simulink model "qpswnymf"  (Simulink 5.0)
settings: Solver=ode45  StartTime=0.0  StopTime=999999  MaxStep=0.05  MinStep=0.000001  RelTol=1e-6  AbsTol=1e-6
values from neighbouring files (symbols this model uses):
  den = real(poly(p(v:v+1)))    [bwthui.m]    (also in rcosfltk.m = 3)
  num = real(poly(z(index)))    [bwthui.m]    (also in rcosfltk.m = 0.5)
undefined symbols (not defined in the file or in its folder): eyediasi, eyesampl, sbiterr
libraries: librnew x1
CloseFcn:
  | closemodcross
settings Model: Creator=gerhard  LastModifiedBy=bauch  ExtModeAutoUpdateStatusClock=off  SaveTime=off  SaveOutput=off  BlockReductionOpt=off  BooleanDataType=off

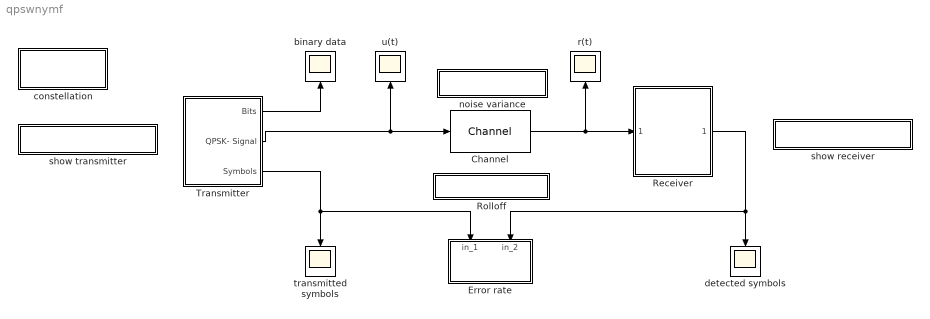
== system qpswnymf ==
  Channel : librnew/Channel  m=0  variance=0.001  s=12345
  Error rate : Subsystem  Orientation=down  LoadFcn=sbiterr([],[],[],'LoadBlock')  StartFcn=sbiterr([],[],[],'Start')  StopFcn=sbiterr([],[],[],'Stop')  mask(Symbol/bit error counter){@1=2, @2=10, @3=12, @4=1}
      mask prompts: @1 "Bit per symbol:"; @2 "Number of digits on display:"; @3 "Delay between 1st port and 2nd port:"; @4 "Sample time (sec):"
      mask help: Use the input data from the 1st port as the reference signal to detect the number of errors and error rate of the 2nd signal.
      mask init:
      | K=@1;num_lin=@2;TDelay=@3;Sample=@4;
      settings: CopyFcn=sbiterr([],[],[],'CopyBlock')  DeleteFcn=sbiterr([],[],[],'DeleteBlock')  NameChangeFcn=sbiterr([],[],[],'NameChange')
      mask Help: The signal from the first port must be a scalar. The second input port can be a vector with a delay to the first port signal. The comparison happens only at the sampling point.
      mask Display: disp('Error\nmeter')
  Receiver : Subsystem
  Rolloff : Subsystem
      settings: OpenFcn=setrloff
      mask Type: rolloff
      mask Display: disp('Rolloff-Factor')
  Transmitter : Subsystem
  binary data : Scope
      settings: Orientation=up  TimeRange=25.000000  YMin=-3  YMax=3  DataFormat=Array
  constellation : Subsystem
      settings: OpenFcn=cplotpsk(4)
      mask Type: constellation
      mask Display: disp('Signal Space \n Constellation')
  detected symbols : Scope
      settings: Orientation=down  TimeRange=25.000000  YMin=-3  YMax=3  DataFormat=Array
  noise variance : Subsystem
      settings: OpenFcn=setnoise
      mask Type: noise
      mask Display: disp('Noise variance')
  r(t) : Scope
      settings: Orientation=up  TimeRange=25.000000  YMin=-1.5  YMax=1.5  DataFormat=Array
  show receiver : Subsystem
      settings: OpenFcn=showrec
      mask Type: open
      mask Display: disp('Receiver')
  show transmitter : Subsystem
      settings: OpenFcn=showtra
      mask Type: open
      mask Display: disp('Transmitter')
  transmitted symbols : Scope
      settings: Orientation=down  TimeRange=25.000000  YMin=-3  YMax=3  DataFormat=Array
  u(t) : Scope
      settings: Orientation=up  TimeRange=25.000000  YMin=-1.5  YMax=1.5  DataFormat=Array
  wires:
  Transmitter/2(QPSK- Signal) -> u(t)/1, Channel/1
  Transmitter/3(Symbols) -> transmitted symbols/1, Error rate/1(in_1)
  Transmitter/1(Bits) -> binary data/1
  Channel/1 -> Receiver/1(noisy QPSK- signal), r(t)/1
  Receiver/1(detected bits) -> detected symbols/1, Error rate/2(in_2)

== system qpswnymf/Error rate ==
  in_1 : Inport
  in_2 : Inport  Port=2
  Mux : Mux  Inputs=2
  S-function : S-Function  FunctionName=sbiterr  Parameters=num_lin, K, TDelay, Sample
  wires:
  Mux/1 -> S-function/1
  in_1/1 -> Mux/1
  in_2/1 -> Mux/2

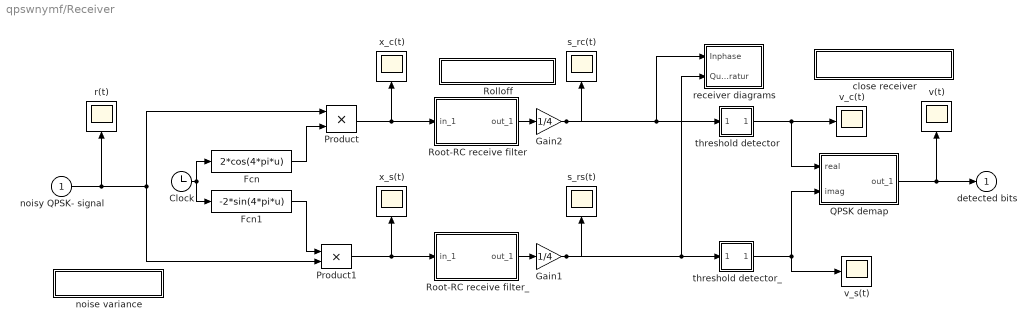
== system qpswnymf/Receiver ==
  noisy QPSK- signal : Inport
  Clock : Clock
      settings: Decimation=10
  Fcn : Fcn  Expr=2*cos(4*pi*u)
  Fcn1 : Fcn  Expr=-2*sin(4*pi*u)
  Gain1 : Gain  Gain=1/4  SaturateOnIntegerOverflow=on
  Gain2 : Gain  Gain=1/4  SaturateOnIntegerOverflow=on
  Product : Product  SaturateOnIntegerOverflow=on  InputSameDT=on
  Product1 : Product  SaturateOnIntegerOverflow=on  InputSameDT=on
  QPSK demap : Subsystem  mask(MPSK demapping){N=[4], A=[sqrt(2)], P=[pi/4], td=1}
      mask prompts: N "Number of symbols on each circle NIC::"; A "Radii for each circle RIC:"; P "Phase shift on each circle PIC (rad):"; td "Symbol interval and offset (sec):"
      mask help:
      | Reverse the QASK map. Input in-phase
      | and quadrature components from the
      | two inputs. Output demapped signal.
      mask init:
      | y1=apkconst(N,A,P);y2=imag(y1);y1=real(y1);
      mask Help: This block demaps a QASK mapped signal using circle constellation. You can place this block after a QAM demodulation block. The circle constellation is defined in NIC, RIC, and PIC. The symbol interval can be a two elements vector with the first element being offset. The default offset is zero. Use function MODMAP to view the constellation.
      mask Display: disp('MPSK\ndemapping')
  Rolloff : Subsystem
      settings: OpenFcn=setrloff
      mask Type: rolloff
      mask Display: disp('Rolloff-Factor')
  Root-RC receive filter : Subsystem  mask(R-C filter){@1=1, @2=.05, @3=.5, @4=6, @5='FIR/Sqrt', @6=0}
      mask prompts: @1 "Symbol interval (sec):"; @2 "Computation sampling time (sec):"; @3 "Filter rolloff factor:"; @4 "Delay step (integer to multiply symbol interval):"; @5 "Filter type (FIR or IIR) / (Normal or Sqrt):"; @6 "With or without sinc filter (1 or 0, suggest 1):"
      mask help: Design a raised cosine filter and use it to filter the input signal.
      mask init:
      | td=@1;if length(td)>1,off=td(2);td=td(1);else,off=0;end;ts=@2;R=@3;delay=@4;fil=@5;[num,den]=rcosine(1/td(1),1/ts(1),fil,R,delay);x=@6/2;
      mask Help: This block designs a raised cosine filter using the specified parameter. The filter is used to filter the input signal. You can optionally use the sinc filter in the filtering computation.
      mask Display: disp('R-C\nfilter')
  Root-RC receive filter_ : Subsystem  mask(R-C filter){@1=1, @2=.05, @3=.5, @4=6, @5='FIR/Sqrt', @6=0}
      mask prompts: @1 "Symbol interval (sec):"; @2 "Computation sampling time (sec):"; @3 "Filter rolloff factor:"; @4 "Delay step (integer to multiply symbol interval):"; @5 "Filter type (FIR or IIR) / (Normal or Sqrt):"; @6 "With or without sinc filter (1 or 0, suggest 1):"
      mask help: Design a raised cosine filter and use it to filter the input signal.
      mask init:
      | td=@1;if length(td)>1,off=td(2);td=td(1);else,off=0;end;ts=@2;R=@3;delay=@4;fil=@5;[num,den]=rcosine(1/td(1),1/ts(1),fil,R,delay);x=@6/2;
      mask Help: This block designs a raised cosine filter using the specified parameter. The filter is used to filter the input signal. You can optionally use the sinc filter in the filtering computation.
      mask Display: disp('R-C\nfilter')
  close receiver : Subsystem
      settings: OpenFcn=closerec
      mask Type: close
      mask Display: disp('close receiver')
  noise variance : Subsystem
      settings: OpenFcn=setnoise
      mask Type: noise
      mask Display: disp('Noise variance')
  r(t) : Scope
      settings: Orientation=up  TimeRange=25.000000  YMin=-1.500000  YMax=1.500000  DataFormat=Array
  receiver diagrams : Subsystem  mask(2D-Diagrams){starttime=12, anzahl=40, offset=0}
      mask prompts: starttime "Plot start time:"; anzahl "Samples per time slot (2*T):"; offset "Decision offset:"
      mask help: Eye pattern, signal space trajectory and scatter plot
      mask init:
      | [x, y] = srcsicon(10);
      mask Display: plot(0,0,100,100,x,y)
  s_rc(t) : Scope
      settings: Orientation=up  TimeRange=25.000000  YMin=-1.500000  YMax=1.500000  DataFormat=Array
  s_rs(t) : Scope
      settings: Orientation=up  TimeRange=25.000000  YMin=-1.500000  YMax=1.500000  DataFormat=Array
  threshold detector : Subsystem
      mask Type: Sign
      mask Description: y = sign(x)
      mask Help: Sign Function:\n\t\t\ty = 1 if x > 0\n\t\t\ty = 0 if x = 0\n\t\t\ty = -1 if x < 0
      mask Display: plot(-50,-50,50,50,[-50,50],[0,0],[0,0],[-50,50],[-40,0],[-30,-30],[0,40],[30,30])
  threshold detector_ : Subsystem
      mask Type: Sign
      mask Description: y = sign(x)
      mask Help: Sign Function:\n\t\t\ty = 1 if x > 0\n\t\t\ty = 0 if x = 0\n\t\t\ty = -1 if x < 0
      mask Display: plot(-50,-50,50,50,[-50,50],[0,0],[0,0],[-50,50],[-40,0],[-30,-30],[0,40],[30,30])
  v(t) : Scope
      settings: Orientation=up  TimeRange=25.000000  YMin=-3.000000  YMax=3.000000  DataFormat=Array
  v_c(t) : Scope
      settings: TimeRange=25.000000  YMin=-1.500000  YMax=1.500000  DataFormat=Array
  v_s(t) : Scope
      settings: TimeRange=25.000000  YMin=-1.500000  YMax=1.500000  DataFormat=Array
  x_c(t) : Scope
      settings: Orientation=up  TimeRange=25.000000  YMin=-1.500000  YMax=1.500000  DataFormat=Array
  x_s(t) : Scope
      settings: Orientation=up  TimeRange=25.000000  YMin=-1.500000  YMax=1.500000  DataFormat=Array
  detected bits : Outport
  wires:
  Clock/1 -> Fcn/1, Fcn1/1
  Product/1 -> Root-RC receive filter/1(in_1), x_c(t)/1
  Product1/1 -> Root-RC receive filter_/1(in_1), x_s(t)/1
  noisy QPSK- signal/1 -> r(t)/1, Product/1, Product1/2
  Fcn1/1 -> Product1/1
  Fcn/1 -> Product/2
  Root-RC receive filter/1(out_1) -> Gain2/1
  Root-RC receive filter_/1(out_1) -> Gain1/1
  Gain2/1 -> s_rc(t)/1, receiver diagrams/1(Inphase), threshold detector/1(in_1)
  Gain1/1 -> s_rs(t)/1, receiver diagrams/2(Quadratur), threshold detector_/1(in_1)
  QPSK demap/1(out_1) -> detected bits/1, v(t)/1
  threshold detector/1(out_1) -> QPSK demap/1(real), v_c(t)/1
  threshold detector_/1(out_1) -> QPSK demap/2(imag), v_s(t)/1

== system qpswnymf/Rolloff ==

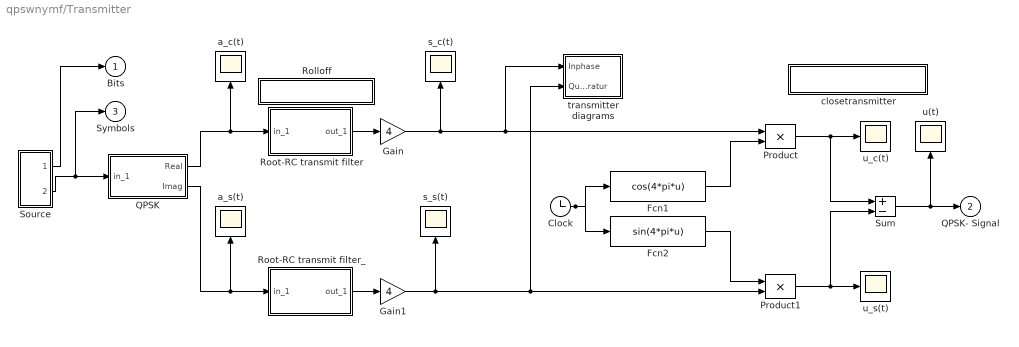
== system qpswnymf/Transmitter ==
  Clock : Clock
      settings: Decimation=10
  Fcn1 : Fcn  Expr=cos(4*pi*u)
  Fcn2 : Fcn  Expr=sin(4*pi*u)
  Gain : Gain  Gain=4  SaturateOnIntegerOverflow=on
  Gain1 : Gain  Gain=4  SaturateOnIntegerOverflow=on
  Product : Product  SaturateOnIntegerOverflow=on  InputSameDT=on
  Product1 : Product  SaturateOnIntegerOverflow=on  InputSameDT=on
  QPSK : Subsystem  mask(MPSK){N=[4], A=[sqrt(2)], P=[pi/4], td=1}
      mask prompts: N "Number of symbols in each circle NIC:"; A "Radii in each circle RIC:"; P "Phase shift in each circle PIC (rad):"; td "Symbol interval and offset (sec):"
      mask help: QASK mapping with circle constellation. The constellation is defined in NIC, RIC and PIC.
      mask init:
      | y1=apkconst(N,A,P);y1=[y1;y1];y1=y1(:);y2=imag(y1);y1=real(y1);x=[-sum(N) 1:sum(N)-1;1:sum(N)-1 10*sum(N)]-.5;x=x(:);
      mask Help: This block maps a digital signal onto in-phase and quadratic components, which are outputs in the first and second output port respectively. The circle constellation is defined in NIC, RIC, and PIC. The input symbol interval can be a two-element vector with the second element being offset. The default value offset is 0. Use the MODMAP function to see the constellation.
      mask Display: disp('MPSK\nmapping')
  Rolloff : Subsystem
      settings: OpenFcn=setrloff
      mask Type: rolloff
      mask Display: disp('Rolloff-Factor')
  Root-RC transmit filter : Subsystem  mask(R-C filter){@1=1, @2=.05, @3=.5, @4=6, @5='FIR/Sqrt', @6=1}
      mask prompts: @1 "Symbol interval (sec):"; @2 "Computation sampling time (sec):"; @3 "Filter rolloff factor:"; @4 "Delay step (integer to multiply symbol interval):"; @5 "Filter type (FIR or IIR) / (Normal or Sqrt):"; @6 "With or without sinc filter (1 or 0, suggest 1):"
      mask help: Design a raised cosine filter and use it to filter the input signal.
      mask init:
      | td=@1;if length(td)>1,off=td(2);td=td(1);else,off=0;end;ts=@2;R=@3;delay=@4;fil=@5;[num,den]=rcosine(1/td(1),1/ts(1),fil,R,delay);x=@6/2;
      mask Help: This block designs a raised cosine filter using the specified parameter. The filter is used to filter the input signal. You can optionally use the sinc filter in the filtering computation.
      mask Display: disp('R-C\nfilter')
  Root-RC transmit filter_ : Subsystem  mask(R-C filter){@1=1, @2=.05, @3=.5, @4=6, @5='FIR/Sqrt', @6=1}
      mask prompts: @1 "Symbol interval (sec):"; @2 "Computation sampling time (sec):"; @3 "Filter rolloff factor:"; @4 "Delay step (integer to multiply symbol interval):"; @5 "Filter type (FIR or IIR) / (Normal or Sqrt):"; @6 "With or without sinc filter (1 or 0, suggest 1):"
      mask help: Design a raised cosine filter and use it to filter the input signal.
      mask init:
      | td=@1;if length(td)>1,off=td(2);td=td(1);else,off=0;end;ts=@2;R=@3;delay=@4;fil=@5;[num,den]=rcosine(1/td(1),1/ts(1),fil,R,delay);x=@6/2;
      mask Help: This block designs a raised cosine filter using the specified parameter. The filter is used to filter the input signal. You can optionally use the sinc filter in the filtering computation.
      mask Display: disp('R-C\nfilter')
  Source : Subsystem
  Sum : Sum  Inputs=+-  SaturateOnIntegerOverflow=on  InputSameDT=on
  a_c(t) : Scope
      settings: Orientation=up  TimeRange=25.000000  YMin=-1.500000  YMax=1.500000  DataFormat=Array
  a_s(t) : Scope
      settings: Orientation=up  TimeRange=25.000000  YMin=-1.500000  YMax=1.500000  DataFormat=Array
  closetransmitter : Subsystem
      settings: OpenFcn=closetra
      mask Type: close
      mask Display: disp('Close transmitter')
  s_c(t) : Scope
      settings: Orientation=up  TimeRange=25.000000  YMin=-1.500000  YMax=1.500000  DataFormat=Array
  s_s(t) : Scope
      settings: Orientation=up  TimeRange=25.000000  YMin=-1.500000  YMax=1.500000  DataFormat=Array
  transmitter diagrams : Subsystem  mask(2D-Diagrams){starttime=6, anzahl=40, offset=0}
      mask prompts: starttime "Plot start time:"; anzahl "Samples per time slot (2*T):"; offset "Decision offset:"
      mask help: Eye pattern, signal space trajectory and scatter plot
      mask init:
      | [x, y] = srcsicon(10);
      mask Display: plot(0,0,100,100,x,y)
  u(t) : Scope
      settings: Orientation=up  TimeRange=25.000000  YMin=-1.500000  YMax=1.500000  DataFormat=Array
  u_c(t) : Scope
      settings: TimeRange=25.000000  YMin=-1.500000  YMax=1.500000  DataFormat=Array
  u_s(t) : Scope
      settings: TimeRange=25.000000  YMin=-1.500000  YMax=1.500000  DataFormat=Array
  Bits : Outport
  QPSK- Signal : Outport  Port=2
  Symbols : Outport  Port=3
  wires:
  QPSK/2(Imag) -> Root-RC transmit filter_/1(in_1), a_s(t)/1
  QPSK/1(Real) -> Root-RC transmit filter/1(in_1), a_c(t)/1
  Source/2(Symbol) -> QPSK/1(in_1), Symbols/1
  Product1/1 -> u_s(t)/1, Sum/2
  Product/1 -> u_c(t)/1, Sum/1
  Gain/1 -> s_c(t)/1, Product/1, transmitter diagrams/1(Inphase)
  Gain1/1 -> s_s(t)/1, Product1/2, transmitter diagrams/2(Quadratur)
  Root-RC transmit filter_/1(out_1) -> Gain1/1
  Root-RC transmit filter/1(out_1) -> Gain/1
  Clock/1 -> Fcn2/1, Fcn1/1
  Fcn1/1 -> Product/2
  Fcn2/1 -> Product1/1
  Sum/1 -> u(t)/1, QPSK- Signal/1
  Source/1(binary) -> Bits/1

== system qpswnymf/constellation ==

== system qpswnymf/noise variance ==

== system qpswnymf/show receiver ==

== system qpswnymf/show transmitter ==

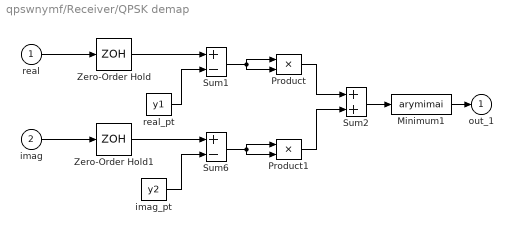
== system qpswnymf/Receiver/QPSK demap ==
  real : Inport
  imag : Inport  Port=2
  Minimum1 : S-Function  FunctionName=arymimai  Parameters='min'
  Product : Product  SaturateOnIntegerOverflow=on  InputSameDT=on
  Product1 : Product  SaturateOnIntegerOverflow=on  InputSameDT=on
  Sum1 : Sum  Inputs=+-  SaturateOnIntegerOverflow=on  InputSameDT=on
  Sum2 : Sum  SaturateOnIntegerOverflow=on  InputSameDT=on
  Sum6 : Sum  Inputs=+-  SaturateOnIntegerOverflow=on  InputSameDT=on
  Zero-Order Hold : ZeroOrderHold  SampleTime=td
  Zero-Order Hold1 : ZeroOrderHold  SampleTime=td
  imag_pt : Constant  Value=y2
  real_pt : Constant  Value=y1
  out_1 : Outport
  wires:
  Minimum1/1 -> out_1/1
  Sum2/1 -> Minimum1/1
  Product1/1 -> Sum2/2
  Product/1 -> Sum2/1
  Sum6/1 -> Product1/2, Product1/1
  Sum1/1 -> Product/2, Product/1
  imag_pt/1 -> Sum6/2
  Zero-Order Hold1/1 -> Sum6/1
  Zero-Order Hold/1 -> Sum1/1
  real_pt/1 -> Sum1/2
  imag/1 -> Zero-Order Hold1/1
  real/1 -> Zero-Order Hold/1

== system qpswnymf/Receiver/Rolloff ==

== system qpswnymf/Receiver/Root-RC receive filter ==
  in_1 : Inport
  Filter : DiscreteFilter  Numerator=num  Denominator=den  SampleTime=ts
  Memory Impulse : Subsystem  mask(Impulse){@1=ts, @2=x}
      mask prompts: @1 "Holding time:"; @2 "Threshold for clock pulse:"
      mask help: 1/sinc filter:
      mask init:
      | ts=@1;thr=@2;x=thr>0;
      mask Help: When the threshold is greater than zero, this block outputs an impulse signal, which begins at the raising edge of the second input and lasts the holding time. The impulse holds a constant amplitude, which equals the amplitude of the first input at the begining of the impulse. A clock raising edge will trigger next impulse. When the threshold is less or equal to zero, this block faithfully outputs the first input.
      mask Display: disp('1/sinc')
  Pulses deivide same sample time1 : Subsystem  mask(Pulse generator){@1=td, @2=1, @3=off}
      mask prompts: @1 "Sample time (scalar, sec):"; @2 "Divider (integer vector):"; @3 "Offset (have same dimension as Divider:"
      mask help: Vector pulses with sample rate of each pulse as Sample_time ./Divider.
      mask init:
      | samp_time=@1;out_divid=@2;offset=@3;
      mask Help: This block generator a vector pulses. The output length is the same as the vector defined in "Divider". The ith element of the output has the sample time Sample_time/Divider(i). All elements in "Divider" must be integers.
      mask Display: disp('Vector\nPulse')
  out_1 : Outport
  wires:
  Pulses deivide same sample time1/1(Outport) -> Memory Impulse/2(in_2)
  Memory Impulse/1(out_1) -> Filter/1
  in_1/1 -> Memory Impulse/1(in_1)
  Filter/1 -> out_1/1

== system qpswnymf/Receiver/Root-RC receive filter_ ==
  in_1 : Inport
  Filter : DiscreteFilter  Numerator=num  Denominator=den  SampleTime=ts
  Memory Impulse : Subsystem  mask(Impulse){@1=ts, @2=x}
      mask prompts: @1 "Holding time:"; @2 "Threshold for clock pulse:"
      mask help: 1/sinc filter:
      mask init:
      | ts=@1;thr=@2;x=thr>0;
      mask Help: When the threshold is greater than zero, this block outputs an impulse signal, which begins at the raising edge of the second input and lasts the holding time. The impulse holds a constant amplitude, which equals the amplitude of the first input at the begining of the impulse. A clock raising edge will trigger next impulse. When the threshold is less or equal to zero, this block faithfully outputs the first input.
      mask Display: disp('1/sinc')
  Pulses deivide same sample time1 : Subsystem  mask(Pulse generator){@1=td, @2=1, @3=off}
      mask prompts: @1 "Sample time (scalar, sec):"; @2 "Divider (integer vector):"; @3 "Offset (have same dimension as Divider:"
      mask help: Vector pulses with sample rate of each pulse as Sample_time ./Divider.
      mask init:
      | samp_time=@1;out_divid=@2;offset=@3;
      mask Help: This block generator a vector pulses. The output length is the same as the vector defined in "Divider". The ith element of the output has the sample time Sample_time/Divider(i). All elements in "Divider" must be integers.
      mask Display: disp('Vector\nPulse')
  out_1 : Outport
  wires:
  Filter/1 -> out_1/1
  in_1/1 -> Memory Impulse/1(in_1)
  Memory Impulse/1(out_1) -> Filter/1
  Pulses deivide same sample time1/1(Outport) -> Memory Impulse/2(in_2)

== system qpswnymf/Receiver/close receiver ==

== system qpswnymf/Receiver/noise variance ==

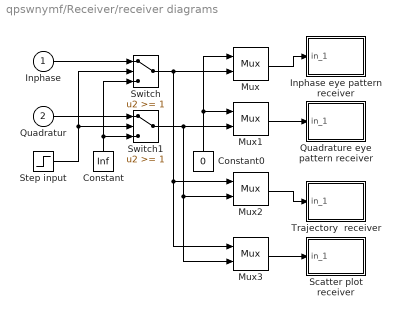
== system qpswnymf/Receiver/receiver diagrams ==
  Inphase : Inport
  Quadratur : Inport  Port=2
  Constant : Constant  Orientation=up  Value=Inf
  Constant0 : Constant  Orientation=up  Value=0
  Inphase eye pattern receiver : Subsystem  LoadFcn=eyesampl([],[],[],'LoadBlock')  StartFcn=eyesampl([],[],[],'Start')  StopFcn=eyesampl([],[],[],'Stop')  mask(Eye-diagram/scatter plot){@1=[2 0 1+offset], @2=[-1.5 1.5], @3=0, @4='w-/r-', @5=0, @6=2/anzahl}
      mask prompts: @1 "[Symbol interval, plot offset, decision point offset]:"; @2 "Lower and upper bound of in-coming signal (1x2 vector):"; @3 "Number of saved traces:"; @4 "Line-type for eye-pattern diagram (0 for no plot):"; @5 "Line-type for scatter plot (0 for no plot):"; @6 "Plot update sample time:"
      mask help: Produce eye-pattern diagram and/or scatter plot.
      mask init:
      | time_range=@1;boundary=@2;kept_length=@3;eye_line=@4;scatter_line=@5;two_d_line=@6;[x,y]=srcsicon(10);
      settings: CopyFcn=eyesampl([],[],[],'CopyBlock')  DeleteFcn=eyesampl([],[],[],'DeleteBlock')  NameChangeFcn=eyesampl([],[],[],'NameChange')
      mask Help: This plot opens one, or two plots by assigning the line type parameters. The scatter plot point is selected by the decision point in the first parameter entry. A decision line is drawn in the eye-pattern diagram. The plot is updated at the plot update sample time point.
      mask Display: plot(0,0,100,100,x,y);
  Mux{,1..3} (4 alike) : Mux  Inputs=2
  Quadrature eye pattern receiver : Subsystem  LoadFcn=eyesampl([],[],[],'LoadBlock')  StartFcn=eyesampl([],[],[],'Start')  StopFcn=eyesampl([],[],[],'Stop')  mask(Eye-diagram/scatter plot){@1=[2 0 1+offset], @2=[-1.5 1.5], @3=0, @4='w-/r-', @5=0, @6=2/anzahl}
      mask prompts: @1 "[Symbol interval, plot offset, decision point offset]:"; @2 "Lower and upper bound of in-coming signal (1x2 vector):"; @3 "Number of saved traces:"; @4 "Line-type for eye-pattern diagram (0 for no plot):"; @5 "Line-type for scatter plot (0 for no plot):"; @6 "Plot update sample time:"
      mask help: Produce eye-pattern diagram and/or scatter plot.
      mask init:
      | time_range=@1;boundary=@2;kept_length=@3;eye_line=@4;scatter_line=@5;two_d_line=@6;[x,y]=srcsicon(10);
      settings: CopyFcn=eyesampl([],[],[],'CopyBlock')  DeleteFcn=eyesampl([],[],[],'DeleteBlock')  NameChangeFcn=eyesampl([],[],[],'NameChange')
      mask Help: This plot opens one, or two plots by assigning the line type parameters. The scatter plot point is selected by the decision point in the first parameter entry. A decision line is drawn in the eye-pattern diagram. The plot is updated at the plot update sample time point.
      mask Display: plot(0,0,100,100,x,y);
  Scatter plot receiver : Subsystem  LoadFcn=eyesampl([],[],[],'LoadBlock')  StartFcn=eyesampl([],[],[],'Start')  StopFcn=eyesampl([],[],[],'Stop')  mask(Eye-diagram/scatter plot){@1=[1 .5 .999], @2=[-1.5 1.5], @3=0, @4=0, @5='b.', @6=[.5 offset]}
      mask prompts: @1 "[Symbol interval, plot offset, decision point offset]:"; @2 "Lower and upper bound of in-coming signal (1x2 vector):"; @3 "Number of saved traces:"; @4 "Line-type for eye-pattern diagram (0 for no plot):"; @5 "Line-type for scatter plot (0 for no plot):"; @6 "Plot update sample time:"
      mask help: Produce eye-pattern diagram and/or scatter plot.
      mask init:
      | time_range=@1;boundary=@2;kept_length=@3;eye_line=@4;scatter_line=@5;two_d_line=@6;[x,y]=srcsicon(10);
      settings: CopyFcn=eyesampl([],[],[],'CopyBlock')  DeleteFcn=eyesampl([],[],[],'DeleteBlock')  NameChangeFcn=eyesampl([],[],[],'NameChange')
      mask Help: This plot opens one, or two plots by assigning the line type parameters. The scatter plot point is selected by the decision point in the first parameter entry. A decision line is drawn in the eye-pattern diagram. The plot is updated at the plot update sample time point.
      mask Display: plot(0,0,100,100,x,y);
  Step input : Step  Time=starttime  SampleTime=1
  Switch : Switch  Threshold=1  SaturateOnIntegerOverflow=on  InputSameDT=on
  Switch1 : Switch  Threshold=1  SaturateOnIntegerOverflow=on  InputSameDT=on
  Trajectory  receiver : Subsystem  LoadFcn=eyediasi([],[],[],'LoadBlock')  StartFcn=eyediasi([],[],[],'Start')  StopFcn=eyediasi([],[],[],'Stop')  mask(Eye-diagram/scatter plot){@1=[2 0 1], @2=[-1.5 1.5], @3=0, @4=0, @5=0, @6='g-'}
      mask prompts: @1 "Eye-pattern plot time frame:"; @2 "Lower and upper bound of in-coming signal (1x2 vector):"; @3 "Number of saved traces:"; @4 "Line-type for eye-pattern diagram (0 for no plot):"; @5 "Line-type for scatter plot (0 for no plot):"; @6 "Line-type for x-y plot (0 for no plot):"
      mask help:
      | Produce eye-pattern diagram/scatter
      | plot/x-y plot with the rising edge of the second input as the decision line.
      mask init:
      | time_range=@1;boundary=@2;kept_length=@3;eye_line=@4;scatter_line=@5;two_d_line=@6;[x,y]=srcsicon(10);[v,w]=trigicon(0,25,get_param(gcb,'orientation'),2);
      settings: CopyFcn=eyediasi([],[],[],'CopyBlock')  DeleteFcn=eyediasi([],[],[],'DeleteBlock')  NameChangeFcn=eyediasi([],[],[],'NameChange')
      mask Help: This plot opens one, two, or three plots by assigning the line type parameters. The scatter plot point is selected by the rising edge of a trigger signal. A decision line is drawn at the rising edge of the trigger signal.
      mask Display: plot(0,0,100,100,x,y,v,w);
  wires:
  Switch/1 -> Mux/2, Mux3/1, Mux2/1
  Switch1/1 -> Mux1/2, Mux3/2, Mux2/2
  Constant0/1 -> Mux1/1, Mux/1
  Quadratur/1 -> Switch1/1
  Inphase/1 -> Switch/1
  Step input/1 -> Switch/2, Switch1/2
  Constant/1 -> Switch/3, Switch1/3
  Mux1/1 -> Quadrature eye pattern receiver/1(in_1)
  Mux/1 -> Inphase eye pattern receiver/1(in_1)
  Mux3/1 -> Scatter plot receiver/1(in_1)
  Mux2/1 -> Trajectory  receiver/1(in_1)

== system qpswnymf/Receiver/threshold detector ==
  in_1 : Inport
  Constant : Constant  Value=0
  Relational Operator : RelationalOperator  Operator=>  InputSameDT=on
  Relational Operator1 : RelationalOperator  Operator=<  InputSameDT=on
  Sum : Sum  Inputs=+-  SaturateOnIntegerOverflow=on  InputSameDT=on
  out_1 : Outport
  wires:
  in_1/1 -> Relational Operator/1, Relational Operator1/1
  Constant/1 -> Relational Operator1/2, Relational Operator/2
  Relational Operator1/1 -> Sum/2
  Relational Operator/1 -> Sum/1
  Sum/1 -> out_1/1

== system qpswnymf/Receiver/threshold detector_ ==
  in_1 : Inport
  Constant : Constant  Value=0
  Relational Operator : RelationalOperator  Operator=>  InputSameDT=on
  Relational Operator1 : RelationalOperator  Operator=<  InputSameDT=on
  Sum : Sum  Inputs=+-  SaturateOnIntegerOverflow=on  InputSameDT=on
  out_1 : Outport
  wires:
  Sum/1 -> out_1/1
  Relational Operator/1 -> Sum/1
  Relational Operator1/1 -> Sum/2
  Constant/1 -> Relational Operator1/2, Relational Operator/2
  in_1/1 -> Relational Operator/1, Relational Operator1/1

== system qpswnymf/Transmitter/QPSK ==
  in_1 : Inport
  Zero-Order Hold1 : ZeroOrderHold  SampleTime=td
  imag part1 : Lookup  InputValues=x  OutputValues=y2  SaturateOnIntegerOverflow=on
  real part : Lookup  InputValues=x  OutputValues=y1  SaturateOnIntegerOverflow=on
  Real : Outport
  Imag : Outport  Port=2
  wires:
  in_1/1 -> Zero-Order Hold1/1
  Zero-Order Hold1/1 -> real part/1, imag part1/1
  real part/1 -> Real/1
  imag part1/1 -> Imag/1

== system qpswnymf/Transmitter/Rolloff ==

== system qpswnymf/Transmitter/Root-RC transmit filter ==
  in_1 : Inport
  Filter : DiscreteFilter  Numerator=num  Denominator=den  SampleTime=ts
  Memory Impulse : Subsystem  mask(Impulse){@1=ts, @2=x}
      mask prompts: @1 "Holding time:"; @2 "Threshold for clock pulse:"
      mask help: 1/sinc filter:
      mask init:
      | ts=@1;thr=@2;x=thr>0;
      mask Help: When the threshold is greater than zero, this block outputs an impulse signal, which begins at the raising edge of the second input and lasts the holding time. The impulse holds a constant amplitude, which equals the amplitude of the first input at the begining of the impulse. A clock raising edge will trigger next impulse. When the threshold is less or equal to zero, this block faithfully outputs the first input.
      mask Display: disp('1/sinc')
  Pulses deivide same sample time1 : Subsystem  mask(Pulse generator){@1=td, @2=1, @3=off}
      mask prompts: @1 "Sample time (scalar, sec):"; @2 "Divider (integer vector):"; @3 "Offset (have same dimension as Divider:"
      mask help: Vector pulses with sample rate of each pulse as Sample_time ./Divider.
      mask init:
      | samp_time=@1;out_divid=@2;offset=@3;
      mask Help: This block generator a vector pulses. The output length is the same as the vector defined in "Divider". The ith element of the output has the sample time Sample_time/Divider(i). All elements in "Divider" must be integers.
      mask Display: disp('Vector\nPulse')
  out_1 : Outport
  wires:
  Pulses deivide same sample time1/1(Outport) -> Memory Impulse/2(in_2)
  Memory Impulse/1(out_1) -> Filter/1
  in_1/1 -> Memory Impulse/1(in_1)
  Filter/1 -> out_1/1

== system qpswnymf/Transmitter/Root-RC transmit filter_ ==
  in_1 : Inport
  Filter : DiscreteFilter  Numerator=num  Denominator=den  SampleTime=ts
  Memory Impulse : Subsystem  mask(Impulse){@1=ts, @2=x}
      mask prompts: @1 "Holding time:"; @2 "Threshold for clock pulse:"
      mask help: 1/sinc filter:
      mask init:
      | ts=@1;thr=@2;x=thr>0;
      mask Help: When the threshold is greater than zero, this block outputs an impulse signal, which begins at the raising edge of the second input and lasts the holding time. The impulse holds a constant amplitude, which equals the amplitude of the first input at the begining of the impulse. A clock raising edge will trigger next impulse. When the threshold is less or equal to zero, this block faithfully outputs the first input.
      mask Display: disp('1/sinc')
  Pulses deivide same sample time1 : Subsystem  mask(Pulse generator){@1=td, @2=1, @3=off}
      mask prompts: @1 "Sample time (scalar, sec):"; @2 "Divider (integer vector):"; @3 "Offset (have same dimension as Divider:"
      mask help: Vector pulses with sample rate of each pulse as Sample_time ./Divider.
      mask init:
      | samp_time=@1;out_divid=@2;offset=@3;
      mask Help: This block generator a vector pulses. The output length is the same as the vector defined in "Divider". The ith element of the output has the sample time Sample_time/Divider(i). All elements in "Divider" must be integers.
      mask Display: disp('Vector\nPulse')
  out_1 : Outport
  wires:
  Pulses deivide same sample time1/1(Outport) -> Memory Impulse/2(in_2)
  Memory Impulse/1(out_1) -> Filter/1
  in_1/1 -> Memory Impulse/1(in_1)
  Filter/1 -> out_1/1

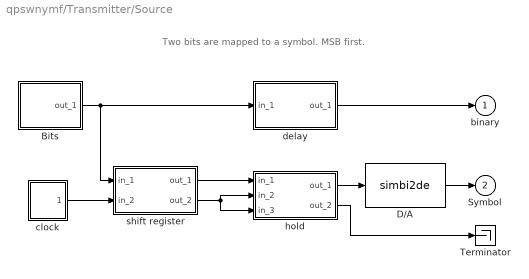
== system qpswnymf/Transmitter/Source ==
  note: Two bits are mapped to a symbol. MSB first.
  Bits : Subsystem  mask(Read from workspace){@1=randint(2000,1,2), @2=.5, @3=1, @4=1}
      mask prompts: @1 "Variable (column_number=block_output_length):"; @2 "Data output sample time (sec):"; @3 "Repeat flag (1: repeat read, 0: output zeros after eof)."; @4 "Initial output:"
      mask help:
      | Read from a workspace variable at
      | sampling time point.
      mask init:
      | var=@1;td=@2;ts=td(1);if (length(td)>=2),off=td(2);else off=0;end;cyc=@3;ini=@4;[x,y]=srcsicon(7);
      mask Help: This block reads from a workspace variable at a given sample time. The column number is the block output vector length. When the simulation reaches the end of the variable (eof), the block will cyclically output from the first row of the variable or output zeros based on the repeat flag entree.
      mask Display: plot(0,0,100,100,x,y);disp('Rd wksp')
  "D/A " : S-Function  FunctionName=simbi2de  Parameters=p  mask(Base M vector to decimal integer){@1=2}
      mask prompts: @1 "Input integer base M:"
      mask help:
      | Convert base M integer with each
      | position in the input vector into scalar decimal output.
      mask init:
      | p=@1;
      mask Help: This block convert the base M vector into scalar decimal integer output. Each element of the input vector is one position of the digit of the base M integer. The 1st element in the input vector contains the 1's position. The 2nd element in the input vector contains the M's position.
      mask Display: disp('Vec to sca\nconverter')
  Terminator : Terminator
  clock : Subsystem  mask(Pulse Generator){@1=.5, @2=.25, @3=1, @4=0}
      mask prompts: @1 "Pulse period (secs):"; @2 "Pulse width:"; @3 "Pulse height:"; @4 "Pulse start time:"
      mask help: Pulse Generator.
      mask init:
      | Ts=@1; du=@2; ht=@3; stt=@4; ini=ones(length(ht),1); st1=rem(stt,Ts); st2=rem(stt+du,Ts);if(Ts<=1.2*du),ini=zeros(length(ht),1);end;
      mask Help: Pulse generator which ensures pulse\ntransitions are hit. Provides a vector of pulses when the height is entered as a vector.\nUnmask to see how it works.
      mask Display: plot(0,0,100,100,[90,75,75,60,60,35,35,20,20,10],[20,20,80,80,20,20,80,80,20,20])
  delay : Subsystem  mask(Multi-step delay){@1=2, @2=.5, @3=0}
      mask prompts: @1 "Delay steps (integer):"; @2 "Sample time (sec):"; @3 "Initial output:"
      mask help: Output is K-step delay of the input signal.
      mask init:
      | n=@1;ts=@2;if length(ts)<2, ts=[ts 0];end;ini=@3;
      mask Help: This block holds the input signal for K steps and then outputs the signal. The delay step cannot be changed during the simulation.
      mask Display: disp('-k\nz   ')
  hold : Subsystem  mask(Triggered buffer down){@1=2, @2=[1 0], @3=[0 0], @4=1, @5=0}
      mask prompts: @1 "Input signal vector size:"; @2 "Initial index (integer vector):"; @3 "Increment for each index (integer vector):"; @4 "Trigger threshold:"; @5 "When index exceed register size, 1: cyclic out, 0: zero out:"
      mask help: Rising edge of the 2nd port triggers 1st port vector signal in. Rising edge of the 3rd port triggers 1st outport signal out.
      mask init:
      | in_size=@1;ini_idx=@2;idx_inc=@3;thrshld=@4;cycl_flag=@5;out_size=length(ini_idx);[v,w]=trigicon(0,25,get_param(gcb,'orientation'),2);[x,y]=trigicon(1,75,get_param(gcb,'orientation'),2);[u,z]=trigicon(0,50,get_param(gcb,'orientation'),2);
      mask Help: The block refreshes its registers with the vector input from the 1st inport at the rising edge of the 2nd inport pulse. The 1st outport outputs the elements of the registers starting with the given initial index. The rising edge of the 3rd inport pulse triggers the 1st output to output the register value with the index increasing the increment value. The second outport outputs a spike pulse when the internal register is refreshed.
      mask Display: plot(0,0,100,100,x,y,v,w,u,z);disp('Buffer dwn')
  shift register : Subsystem  mask(Register-shift){@1=[2 1], @2=1}
      mask prompts: @1 "Delay steps (output length is same as this vector size):"; @2 "Threshold in detecting the rising edge of the pulse:"
      mask help:
      | The rising edge of the 2nd port pulse
      | triggers the block to input the 1st port data and to shift the register.
      mask init:
      | shft_out=@1;thrhld=@2;len_rg=length(@1);[v,w]=trigicon(0,25,get_param(gcb,'orientation'),2);[x,y]=trigicon(1,75,get_param(gcb,'orientation'),2);
      mask Help: This block stores the scalar input signal from the 1st input port at the rising edge of the pulse from the 2nd port. The 1st outport outputs a vector with its size the same as the "Delay steps" entree of this block. The maximum delay is the register size of this block. The second outport outputs a positive pulse when the register is\nrefreshed.
      mask Display: plot(0,0,100,100,x,y,v,w);disp('Reg. shift')
  binary : Outport
  Symbol : Outport  Port=2
  wires:
  hold/2(out_2) -> Terminator/1
  "D/A "/1 -> Symbol/1
  delay/1(out_1) -> binary/1
  shift register/1(out_1) -> hold/1(in_1)
  hold/1(out_1) -> "D/A "/1
  clock/1(out_1) -> shift register/2(in_2)
  shift register/2(out_2) -> hold/2(in_2), hold/3(in_3)
  Bits/1(out_1) -> delay/1(in_1), shift register/1(in_1)

== system qpswnymf/Transmitter/closetransmitter ==

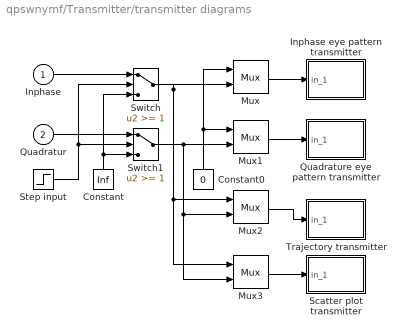
== system qpswnymf/Transmitter/transmitter diagrams ==
  Inphase : Inport
  Quadratur : Inport  Port=2
  Constant : Constant  Orientation=up  Value=Inf
  Constant0 : Constant  Orientation=up  Value=0
  Inphase eye pattern transmitter : Subsystem  LoadFcn=eyesampl([],[],[],'LoadBlock')  StartFcn=eyesampl([],[],[],'Start')  StopFcn=eyesampl([],[],[],'Stop')  mask(Eye-diagram/scatter plot){@1=[2 0 1+offset], @2=[-1.5 1.5], @3=0, @4='w-/r-', @5=0, @6=2/anzahl}
      mask prompts: @1 "[Symbol interval, plot offset, decision point offset]:"; @2 "Lower and upper bound of in-coming signal (1x2 vector):"; @3 "Number of saved traces:"; @4 "Line-type for eye-pattern diagram (0 for no plot):"; @5 "Line-type for scatter plot (0 for no plot):"; @6 "Plot update sample time:"
      mask help: Produce eye-pattern diagram and/or scatter plot.
      mask init:
      | time_range=@1;boundary=@2;kept_length=@3;eye_line=@4;scatter_line=@5;two_d_line=@6;[x,y]=srcsicon(10);
      settings: CopyFcn=eyesampl([],[],[],'CopyBlock')  DeleteFcn=eyesampl([],[],[],'DeleteBlock')  NameChangeFcn=eyesampl([],[],[],'NameChange')
      mask Help: This plot opens one, or two plots by assigning the line type parameters. The scatter plot point is selected by the decision point in the first parameter entry. A decision line is drawn in the eye-pattern diagram. The plot is updated at the plot update sample time point.
      mask Display: plot(0,0,100,100,x,y);
  Mux{,1..3} (4 alike) : Mux  Inputs=2
  Quadrature eye pattern transmitter : Subsystem  LoadFcn=eyesampl([],[],[],'LoadBlock')  StartFcn=eyesampl([],[],[],'Start')  StopFcn=eyesampl([],[],[],'Stop')  mask(Eye-diagram/scatter plot){@1=[2 0 1+offset], @2=[-1.5 1.5], @3=0, @4='w-/r-', @5=0, @6=2/anzahl}
      mask prompts: @1 "[Symbol interval, plot offset, decision point offset]:"; @2 "Lower and upper bound of in-coming signal (1x2 vector):"; @3 "Number of saved traces:"; @4 "Line-type for eye-pattern diagram (0 for no plot):"; @5 "Line-type for scatter plot (0 for no plot):"; @6 "Plot update sample time:"
      mask help: Produce eye-pattern diagram and/or scatter plot.
      mask init:
      | time_range=@1;boundary=@2;kept_length=@3;eye_line=@4;scatter_line=@5;two_d_line=@6;[x,y]=srcsicon(10);
      settings: CopyFcn=eyesampl([],[],[],'CopyBlock')  DeleteFcn=eyesampl([],[],[],'DeleteBlock')  NameChangeFcn=eyesampl([],[],[],'NameChange')
      mask Help: This plot opens one, or two plots by assigning the line type parameters. The scatter plot point is selected by the decision point in the first parameter entry. A decision line is drawn in the eye-pattern diagram. The plot is updated at the plot update sample time point.
      mask Display: plot(0,0,100,100,x,y);
  Scatter plot transmitter : Subsystem  LoadFcn=eyesampl([],[],[],'LoadBlock')  StartFcn=eyesampl([],[],[],'Start')  StopFcn=eyesampl([],[],[],'Stop')  mask(Eye-diagram/scatter plot){@1=[1 .5 .999], @2=[-1.5 1.5], @3=0, @4=0, @5='b.', @6=[.5 offset]}
      mask prompts: @1 "[Symbol interval, plot offset, decision point offset]:"; @2 "Lower and upper bound of in-coming signal (1x2 vector):"; @3 "Number of saved traces:"; @4 "Line-type for eye-pattern diagram (0 for no plot):"; @5 "Line-type for scatter plot (0 for no plot):"; @6 "Plot update sample time:"
      mask help: Produce eye-pattern diagram and/or scatter plot.
      mask init:
      | time_range=@1;boundary=@2;kept_length=@3;eye_line=@4;scatter_line=@5;two_d_line=@6;[x,y]=srcsicon(10);
      settings: CopyFcn=eyesampl([],[],[],'CopyBlock')  DeleteFcn=eyesampl([],[],[],'DeleteBlock')  NameChangeFcn=eyesampl([],[],[],'NameChange')
      mask Help: This plot opens one, or two plots by assigning the line type parameters. The scatter plot point is selected by the decision point in the first parameter entry. A decision line is drawn in the eye-pattern diagram. The plot is updated at the plot update sample time point.
      mask Display: plot(0,0,100,100,x,y);
  Step input : Step  Time=starttime  SampleTime=1
  Switch : Switch  Threshold=1  SaturateOnIntegerOverflow=on  InputSameDT=on
  Switch1 : Switch  Threshold=1  SaturateOnIntegerOverflow=on  InputSameDT=on
  Trajectory transmitter : Subsystem  LoadFcn=eyediasi([],[],[],'LoadBlock')  StartFcn=eyediasi([],[],[],'Start')  StopFcn=eyediasi([],[],[],'Stop')  mask(Eye-diagram/scatter plot){@1=[2 0 1], @2=[-1.5 1.5], @3=0, @4=0, @5=0, @6='g-'}
      mask prompts: @1 "Eye-pattern plot time frame:"; @2 "Lower and upper bound of in-coming signal (1x2 vector):"; @3 "Number of saved traces:"; @4 "Line-type for eye-pattern diagram (0 for no plot):"; @5 "Line-type for scatter plot (0 for no plot):"; @6 "Line-type for x-y plot (0 for no plot):"
      mask help:
      | Produce eye-pattern diagram/scatter
      | plot/x-y plot with the rising edge of the second input as the decision line.
      mask init:
      | time_range=@1;boundary=@2;kept_length=@3;eye_line=@4;scatter_line=@5;two_d_line=@6;[x,y]=srcsicon(10);[v,w]=trigicon(0,25,get_param(gcb,'orientation'),2);
      settings: CopyFcn=eyediasi([],[],[],'CopyBlock')  DeleteFcn=eyediasi([],[],[],'DeleteBlock')  NameChangeFcn=eyediasi([],[],[],'NameChange')
      mask Help: This plot opens one, two, or three plots by assigning the line type parameters. The scatter plot point is selected by the rising edge of a trigger signal. A decision line is drawn at the rising edge of the trigger signal.
      mask Display: plot(0,0,100,100,x,y,v,w);
  wires:
  Mux2/1 -> Trajectory transmitter/1(in_1)
  Mux3/1 -> Scatter plot transmitter/1(in_1)
  Mux/1 -> Inphase eye pattern transmitter/1(in_1)
  Mux1/1 -> Quadrature eye pattern transmitter/1(in_1)
  Constant/1 -> Switch/3, Switch1/3
  Step input/1 -> Switch/2, Switch1/2
  Inphase/1 -> Switch/1
  Quadratur/1 -> Switch1/1
  Switch/1 -> Mux3/1, Mux2/1, Mux/2
  Switch1/1 -> Mux3/2, Mux2/2, Mux1/2
  Constant0/1 -> Mux1/1, Mux/1

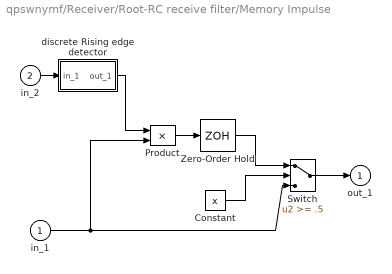
== system qpswnymf/Receiver/Root-RC receive filter/Memory Impulse ==
  in_1 : Inport
  in_2 : Inport  Port=2
  Constant : Constant  Value=x
  Product : Product  SaturateOnIntegerOverflow=on  InputSameDT=on
  Switch : Switch  Threshold=.5  SaturateOnIntegerOverflow=on  InputSameDT=on
  Zero-Order Hold : ZeroOrderHold  SampleTime=ts
  discrete Rising edge detector : Subsystem  mask(Edge Detection){@1=thr, @2=ts}
      mask prompts: @1 "Threshold:"; @2 "Sampling time:"
      mask help: Rising edge detection:
      mask init:
      | thld=@1;ts=@2;
      mask Help: When the input signal rising edge passed the given shreshold, this block outputs one, otherwise outputs zero.
      mask Display: disp('Edge\nDetector')
  out_1 : Outport
  wires:
  Zero-Order Hold/1 -> Switch/1
  Product/1 -> Zero-Order Hold/1
  in_1/1 -> Switch/3, Product/2
  Switch/1 -> out_1/1
  Constant/1 -> Switch/2
  discrete Rising edge detector/1(out_1) -> Product/1
  in_2/1 -> discrete Rising edge detector/1(in_1)

== system qpswnymf/Receiver/Root-RC receive filter/Pulses deivide same sample time1 ==
  S-function1 : S-Function  FunctionName=homopuls  Parameters=samp_time, out_divid, offset
  Outport : Outport
  wires:
  S-function1/1 -> Outport/1

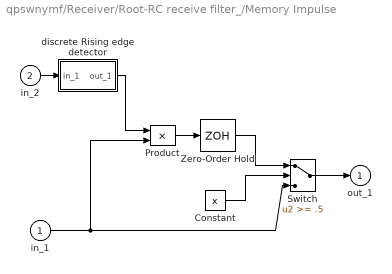
== system qpswnymf/Receiver/Root-RC receive filter_/Memory Impulse ==
  in_1 : Inport
  in_2 : Inport  Port=2
  Constant : Constant  Value=x
  Product : Product  SaturateOnIntegerOverflow=on  InputSameDT=on
  Switch : Switch  Threshold=.5  SaturateOnIntegerOverflow=on  InputSameDT=on
  Zero-Order Hold : ZeroOrderHold  SampleTime=ts
  discrete Rising edge detector : Subsystem  mask(Edge Detection){@1=thr, @2=ts}
      mask prompts: @1 "Threshold:"; @2 "Sampling time:"
      mask help: Rising edge detection:
      mask init:
      | thld=@1;ts=@2;
      mask Help: When the input signal rising edge passed the given shreshold, this block outputs one, otherwise outputs zero.
      mask Display: disp('Edge\nDetector')
  out_1 : Outport
  wires:
  in_2/1 -> discrete Rising edge detector/1(in_1)
  discrete Rising edge detector/1(out_1) -> Product/1
  Constant/1 -> Switch/2
  Switch/1 -> out_1/1
  in_1/1 -> Switch/3, Product/2
  Product/1 -> Zero-Order Hold/1
  Zero-Order Hold/1 -> Switch/1

== system qpswnymf/Receiver/Root-RC receive filter_/Pulses deivide same sample time1 ==
  S-function1 : S-Function  FunctionName=homopuls  Parameters=samp_time, out_divid, offset
  Outport : Outport
  wires:
  S-function1/1 -> Outport/1

== system qpswnymf/Receiver/receiver diagrams/Inphase eye pattern receiver ==
  in_1 : Inport
  Plot1 : S-Function  FunctionName=eyesampl  Parameters=time_range, boundary, kept_length, eye_line, scatter_line, two_d_line
  wires:
  in_1/1 -> Plot1/1

== system qpswnymf/Receiver/receiver diagrams/Quadrature eye pattern receiver ==
  in_1 : Inport
  Plot1 : S-Function  FunctionName=eyesampl  Parameters=time_range, boundary, kept_length, eye_line, scatter_line, two_d_line
  wires:
  in_1/1 -> Plot1/1

== system qpswnymf/Receiver/receiver diagrams/Scatter plot receiver ==
  in_1 : Inport
  Plot1 : S-Function  FunctionName=eyesampl  Parameters=time_range, boundary, kept_length, eye_line, scatter_line, two_d_line
  wires:
  in_1/1 -> Plot1/1

== system qpswnymf/Receiver/receiver diagrams/Trajectory  receiver ==
  in_1 : Inport
  Constant : Constant  Value=0
  Mux : Mux  Inputs=2
  Plot1 : S-Function  FunctionName=eyediasi  Parameters=time_range, boundary, kept_length, eye_line, scatter_line, two_d_line
  wires:
  in_1/1 -> Mux/1
  Constant/1 -> Mux/2
  Mux/1 -> Plot1/1

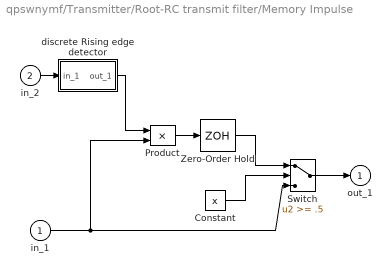
== system qpswnymf/Transmitter/Root-RC transmit filter/Memory Impulse ==
  in_1 : Inport
  in_2 : Inport  Port=2
  Constant : Constant  Value=x
  Product : Product  SaturateOnIntegerOverflow=on  InputSameDT=on
  Switch : Switch  Threshold=.5  SaturateOnIntegerOverflow=on  InputSameDT=on
  Zero-Order Hold : ZeroOrderHold  SampleTime=ts
  discrete Rising edge detector : Subsystem  mask(Edge Detection){@1=thr, @2=ts}
      mask prompts: @1 "Threshold:"; @2 "Sampling time:"
      mask help: Rising edge detection:
      mask init:
      | thld=@1;ts=@2;
      mask Help: When the input signal rising edge passed the given shreshold, this block outputs one, otherwise outputs zero.
      mask Display: disp('Edge\nDetector')
  out_1 : Outport
  wires:
  Zero-Order Hold/1 -> Switch/1
  Product/1 -> Zero-Order Hold/1
  in_1/1 -> Switch/3, Product/2
  Switch/1 -> out_1/1
  Constant/1 -> Switch/2
  discrete Rising edge detector/1(out_1) -> Product/1
  in_2/1 -> discrete Rising edge detector/1(in_1)

== system qpswnymf/Transmitter/Root-RC transmit filter/Pulses deivide same sample time1 ==
  S-function1 : S-Function  FunctionName=homopuls  Parameters=samp_time, out_divid, offset
  Outport : Outport
  wires:
  S-function1/1 -> Outport/1

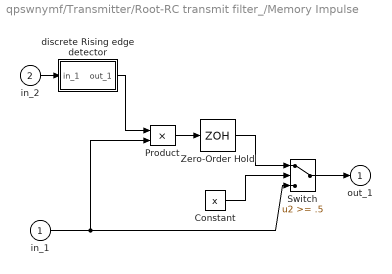
== system qpswnymf/Transmitter/Root-RC transmit filter_/Memory Impulse ==
  in_1 : Inport
  in_2 : Inport  Port=2
  Constant : Constant  Value=x
  Product : Product  SaturateOnIntegerOverflow=on  InputSameDT=on
  Switch : Switch  Threshold=.5  SaturateOnIntegerOverflow=on  InputSameDT=on
  Zero-Order Hold : ZeroOrderHold  SampleTime=ts
  discrete Rising edge detector : Subsystem  mask(Edge Detection){@1=thr, @2=ts}
      mask prompts: @1 "Threshold:"; @2 "Sampling time:"
      mask help: Rising edge detection:
      mask init:
      | thld=@1;ts=@2;
      mask Help: When the input signal rising edge passed the given shreshold, this block outputs one, otherwise outputs zero.
      mask Display: disp('Edge\nDetector')
  out_1 : Outport
  wires:
  Zero-Order Hold/1 -> Switch/1
  Product/1 -> Zero-Order Hold/1
  in_1/1 -> Switch/3, Product/2
  Switch/1 -> out_1/1
  Constant/1 -> Switch/2
  discrete Rising edge detector/1(out_1) -> Product/1
  in_2/1 -> discrete Rising edge detector/1(in_1)

== system qpswnymf/Transmitter/Root-RC transmit filter_/Pulses deivide same sample time1 ==
  S-function1 : S-Function  FunctionName=homopuls  Parameters=samp_time, out_divid, offset
  Outport : Outport
  wires:
  S-function1/1 -> Outport/1

== system qpswnymf/Transmitter/Source/Bits ==
  Message source : S-Function  FunctionName=trigwksp  Parameters=var,thd,cyclFlag,ini  mask(Read from workspace){@1=var, @2=.1, @3=cyc, @4=ini}
      mask prompts: @1 "Read the variable:"; @2 "Threshold for the input pulse:"; @3 "Cyclic read variable (1) or amend zeros (0)."; @4 "Output before first trigger:"
      mask help: The raising edge of input pulse trigger the block output the next row from the workspace variable.
      mask init:
      | var=@1;thd=@2;cyclFlag=@3;ini=@4;
      mask Help: This block reads the data from a workspace variable. The output is refreshed at the raising edge of the input pulse.
      mask Display: disp('Triggered\nread')
  Pulses deivide same sample time1 : Subsystem  mask(Pulse generator){@1=ts, @2=1, @3=off}
      mask prompts: @1 "Sample time (scalar, sec):"; @2 "Divider (integer vector):"; @3 "Offset (have same dimension as Divider:"
      mask help: Vector pulses with sample rate of each pulse as Sample_time ./Divider.
      mask init:
      | samp_time=@1;out_divid=@2;offset=@3;
      mask Help: This block generator a vector pulses. The output length is the same as the vector defined in "Divider". The ith element of the output has the sample time Sample_time/Divider(i). All elements in "Divider" must be integers.
      mask Display: disp('Vector\nPulse')
  out_1 : Outport
  wires:
  Message source/1 -> out_1/1
  Pulses deivide same sample time1/1(Outport) -> Message source/1

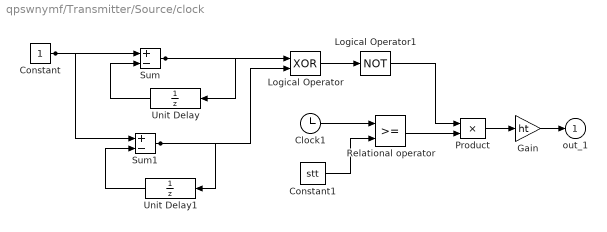
== system qpswnymf/Transmitter/Source/clock ==
  Clock1 : Clock
      settings: Decimation=10
  Constant : Constant
  Constant1 : Constant  Value=stt
  Gain : Gain  Gain=ht  SaturateOnIntegerOverflow=on
  Logical Operator : Logic  Operator=XOR
  Logical Operator1 : Logic  Operator=NOT  Inputs=1
  Product : Product  SaturateOnIntegerOverflow=on  InputSameDT=on
  Relational operator : RelationalOperator  InputSameDT=on
  Sum : Sum  Inputs=+-  SaturateOnIntegerOverflow=on  InputSameDT=on
  Sum1 : Sum  Inputs=+-  SaturateOnIntegerOverflow=on  InputSameDT=on
  Unit Delay : UnitDelay  Orientation=left  SampleTime=[Ts,st1]
  Unit Delay1 : UnitDelay  Orientation=left  X0=ini  SampleTime=[Ts,st2]
  out_1 : Outport
  wires:
  Sum1/1 -> Logical Operator/2, Unit Delay1/1
  Sum/1 -> Logical Operator/1, Unit Delay/1
  Constant/1 -> Sum1/1, Sum/1
  Unit Delay1/1 -> Sum1/2
  Unit Delay/1 -> Sum/2
  Clock1/1 -> Relational operator/1
  Relational operator/1 -> Product/2
  Product/1 -> Gain/1
  Gain/1 -> out_1/1
  Constant1/1 -> Relational operator/2
  Logical Operator/1 -> Logical Operator1/1
  Logical Operator1/1 -> Product/1

== system qpswnymf/Transmitter/Source/delay ==
  in_1 : Inport
  Constant : Constant  Value=ini
  Constant1 : Constant  Value=n*ts(1)+ts(2)
  Digital Clock : DigitalClock  SampleTime=ts
  K-step delay : DiscreteFilter  Numerator=[zeros(1,n), 1]  Denominator=1  SampleTime=ts
  Relational Operator : RelationalOperator  InputSameDT=on
  Switch : Switch  Threshold=.1  SaturateOnIntegerOverflow=on  InputSameDT=on
  out_1 : Outport
  wires:
  Relational Operator/1 -> Switch/2
  Constant1/1 -> Relational Operator/2
  Digital Clock/1 -> Relational Operator/1
  Constant/1 -> Switch/3
  K-step delay/1 -> Switch/1
  in_1/1 -> K-step delay/1
  Switch/1 -> out_1/1

== system qpswnymf/Transmitter/Source/hold ==
  in_1 : Inport
  in_2 : Inport  Port=2
  in_3 : Inport  Port=3
  Demux : Demux  Outputs=[out_size 1]
  Mux : Mux  Inputs=[in_size 1 1]
  S-function : S-Function  FunctionName=regdown  Parameters=ini_idx, idx_inc, thrshld, cycl_flag
  out_1 : Outport
  out_2 : Outport  Port=2
  wires:
  in_3/1 -> Mux/3
  Demux/2 -> out_2/1
  in_2/1 -> Mux/2
  Demux/1 -> out_1/1
  in_1/1 -> Mux/1
  Mux/1 -> S-function/1
  S-function/1 -> Demux/1

== system qpswnymf/Transmitter/Source/shift register ==
  in_1 : Inport
  in_2 : Inport  Port=2
  Demux : Demux  Outputs=[len_rg, 1]
  Mux : Mux  Inputs=2
  S-function : S-Function  FunctionName=regshift  Parameters=shft_out, thrhld
  out_1 : Outport
  out_2 : Outport  Port=2
  wires:
  Mux/1 -> S-function/1
  S-function/1 -> Demux/1
  Demux/1 -> out_1/1
  Demux/2 -> out_2/1
  in_1/1 -> Mux/1
  in_2/1 -> Mux/2

== system qpswnymf/Transmitter/transmitter diagrams/Inphase eye pattern transmitter ==
  in_1 : Inport
  Plot1 : S-Function  FunctionName=eyesampl  Parameters=time_range, boundary, kept_length, eye_line, scatter_line, two_d_line
  wires:
  in_1/1 -> Plot1/1

== system qpswnymf/Transmitter/transmitter diagrams/Quadrature eye pattern transmitter ==
  in_1 : Inport
  Plot1 : S-Function  FunctionName=eyesampl  Parameters=time_range, boundary, kept_length, eye_line, scatter_line, two_d_line
  wires:
  in_1/1 -> Plot1/1

== system qpswnymf/Transmitter/transmitter diagrams/Scatter plot transmitter ==
  in_1 : Inport
  Plot1 : S-Function  FunctionName=eyesampl  Parameters=time_range, boundary, kept_length, eye_line, scatter_line, two_d_line
  wires:
  in_1/1 -> Plot1/1

== system qpswnymf/Transmitter/transmitter diagrams/Trajectory transmitter ==
  in_1 : Inport
  Constant : Constant  Value=0
  Mux : Mux  Inputs=2
  Plot1 : S-Function  FunctionName=eyediasi  Parameters=time_range, boundary, kept_length, eye_line, scatter_line, two_d_line
  wires:
  Mux/1 -> Plot1/1
  Constant/1 -> Mux/2
  in_1/1 -> Mux/1

== system qpswnymf/Receiver/Root-RC receive filter/Memory Impulse/discrete Rising edge detector ==
  in_1 : Inport
  Relational Operator : RelationalOperator  InputSameDT=on
  Relational Operator1 : RelationalOperator  InputSameDT=on
  Relational Operator2 : RelationalOperator  Operator=>  InputSameDT=on
  Unit Delay : UnitDelay  SampleTime=ts
  one1 : Constant  Value=thld
  out_1 : Outport
  wires:
  Relational Operator2/1 -> out_1/1
  Relational Operator1/1 -> Relational Operator2/2
  Relational Operator/1 -> Relational Operator2/1
  one1/1 -> Relational Operator/2, Relational Operator1/2
  Unit Delay/1 -> Relational Operator1/1
  in_1/1 -> Relational Operator/1, Unit Delay/1

== system qpswnymf/Receiver/Root-RC receive filter_/Memory Impulse/discrete Rising edge detector ==
  in_1 : Inport
  Relational Operator : RelationalOperator  InputSameDT=on
  Relational Operator1 : RelationalOperator  InputSameDT=on
  Relational Operator2 : RelationalOperator  Operator=>  InputSameDT=on
  Unit Delay : UnitDelay  SampleTime=ts
  one1 : Constant  Value=thld
  out_1 : Outport
  wires:
  in_1/1 -> Relational Operator/1, Unit Delay/1
  Unit Delay/1 -> Relational Operator1/1
  one1/1 -> Relational Operator/2, Relational Operator1/2
  Relational Operator/1 -> Relational Operator2/1
  Relational Operator1/1 -> Relational Operator2/2
  Relational Operator2/1 -> out_1/1

== system qpswnymf/Transmitter/Root-RC transmit filter/Memory Impulse/discrete Rising edge detector ==
  in_1 : Inport
  Relational Operator : RelationalOperator  InputSameDT=on
  Relational Operator1 : RelationalOperator  InputSameDT=on
  Relational Operator2 : RelationalOperator  Operator=>  InputSameDT=on
  Unit Delay : UnitDelay  SampleTime=ts
  one1 : Constant  Value=thld
  out_1 : Outport
  wires:
  Relational Operator2/1 -> out_1/1
  Relational Operator1/1 -> Relational Operator2/2
  Relational Operator/1 -> Relational Operator2/1
  one1/1 -> Relational Operator/2, Relational Operator1/2
  Unit Delay/1 -> Relational Operator1/1
  in_1/1 -> Relational Operator/1, Unit Delay/1

== system qpswnymf/Transmitter/Root-RC transmit filter_/Memory Impulse/discrete Rising edge detector ==
  in_1 : Inport
  Relational Operator : RelationalOperator  InputSameDT=on
  Relational Operator1 : RelationalOperator  InputSameDT=on
  Relational Operator2 : RelationalOperator  Operator=>  InputSameDT=on
  Unit Delay : UnitDelay  SampleTime=ts
  one1 : Constant  Value=thld
  out_1 : Outport
  wires:
  Relational Operator2/1 -> out_1/1
  Relational Operator1/1 -> Relational Operator2/2
  Relational Operator/1 -> Relational Operator2/1
  one1/1 -> Relational Operator/2, Relational Operator1/2
  Unit Delay/1 -> Relational Operator1/1
  in_1/1 -> Relational Operator/1, Unit Delay/1

== system qpswnymf/Transmitter/Source/Bits/Pulses deivide same sample time1 ==
  S-function1 : S-Function  FunctionName=homopuls  Parameters=samp_time, out_divid, offset
  Outport : Outport
  wires:
  S-function1/1 -> Outport/1
